simulink model "Current"  (R2021a)
settings: Solver=VariableStepAuto  StartTime=0.0  StopTime=10.0  RelTol=1e-3
settings Model: Creator=Admin  LastModifiedBy=Admin

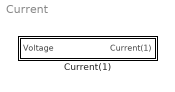
== system Current ==
  Current(1) : Subsystem

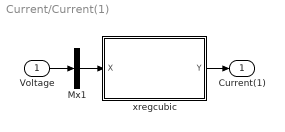
== system Current/Current(1) ==
  Voltage : Inport  Unit=Volts
  Mx1 : Mux  Inputs=1
  xregcubic : Subsystem
      mask init:
      | xregmaskinitialization;
  Current(1) : Outport  Unit=Amps
  wires:
  Voltage/1 -> Mx1/1
  Mx1/1 -> xregcubic/1(X)
  xregcubic/1(Y) -> Current(1)/1

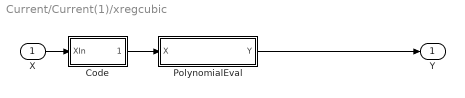
== system Current/Current(1)/xregcubic ==
  X : Inport
  Code : Subsystem
  PolynomialEval : Subsystem
  Y : Outport
  wires:
  X/1 -> Code/1(XIn)
  Code/1(XCoded) -> PolynomialEval/1(X)
  PolynomialEval/1(Y) -> Y/1

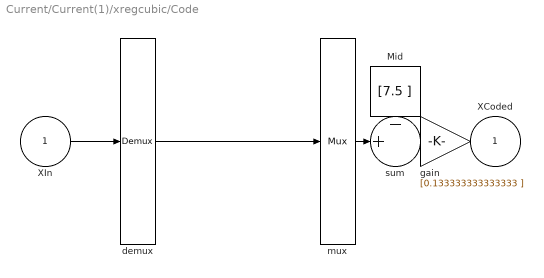
== system Current/Current(1)/xregcubic/Code ==
  XIn : Inport
  Mid : Constant  Value=[7.5 ]
  demux : Demux  Outputs=1
  gain : Gain  Gain=[0.133333333333333 ]
  mux : Mux  Inputs=1
  sum : Sum  Inputs=-+|
  XCoded : Outport
  wires:
  demux/1 -> mux/1
  Mid/1 -> sum/1
  XIn/1 -> demux/1
  mux/1 -> sum/2
  sum/1 -> gain/1
  gain/1 -> XCoded/1

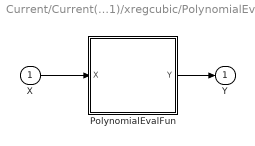
== system Current/Current(1)/xregcubic/PolynomialEval ==
  X : Inport
  PolynomialEvalFun : MATLAB Function  TreatAsAtomicUnit=on
  Y : Outport
  wires:
  X/1 -> PolynomialEvalFun/1(X)
  PolynomialEvalFun/1(Y) -> Y/1

== matlab function Current/Current(1)/xregcubic/PolynomialEval/PolynomialEvalFun ==
  data: X input size=nfactors; Y output; coeffs parameter
function Y = fcn(X, coeffs)
%#codegen

% This function specifies a polynomial with 1 inputs: 
% 	Voltage	 = order 3
% Maximum interaction order = 3
%
% The model definition is:
% 0.72328 + 0.31123*Voltage-0.15354*Voltage^2 + 0.14901*Voltage^3

% Autogenerated by the Model-Based Calibration Toolbox on 14-Dec-2023 10:21:36.


Y = coeffs(1) + X(1)*(coeffs(2) + X(1)*(coeffs(3) + X(1)*coeffs(4)));
